simulink model "Soru4Gorev3"  (R2019a)
settings: Solver=VariableStepAuto  StartTime=0.0  StopTime=10.0  RelTol=1e-3
libraries: simulink x1
settings Model: Creator=handeyildirim  LastModifiedBy=handeyildirim

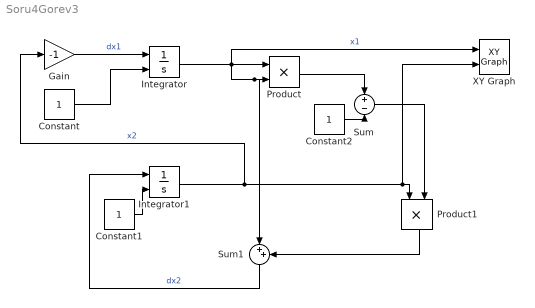
== system Soru4Gorev3 ==
  Constant : Constant
  Constant1 : Constant
  Constant2 : Constant
  Gain : Gain  Gain=-1
  Integrator : Integrator  InitialConditionSource=external
  Integrator1 : Integrator  InitialConditionSource=external
  Product : Product
  Product1 : Product
  Sum : Sum  Inputs=+-
  Sum1 : Sum  Inputs=|++
  XY Graph : simulink/Sinks/XY Graph  xmin=-0.6  xmax=1  ymin=-0.4  ymax=1.2  st=-1
  wires:
  Gain/1 -> Integrator/1  "dx1"
  Constant/1 -> Integrator/2
  Integrator/1 -> XY Graph/1, Sum1/1, Product/2, Product/1  "x1"
  Constant1/1 -> Integrator1/2
  Integrator1/1 -> Gain/1, XY Graph/2, Product1/1  "x2"
  Product/1 -> Sum/1
  Constant2/1 -> Sum/2
  Sum/1 -> Product1/2
  Product1/1 -> Sum1/2
  Sum1/1 -> Integrator1/1  "dx2"
